simulink model "grabber"  (Simulink 6.4)
settings: Solver=ode45  StartTime=0.0  StopTime=inf  RelTol=1e-3
libraries: vipsnks x1, imaqlib x1
settings Model: LastModifiedBy=usman

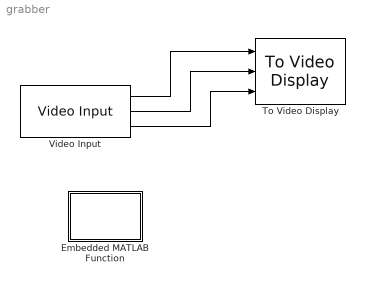
== system grabber ==
  Embedded MATLAB Function : Stateflow chart
  To Video Display : vipsnks/To Video Display  inputType=RGB  OutputDevice=On-screen video monitor  fullScreen=off  videoWindowX=44  videoWindowY=38  saveWindowSize=off  videoWindowWidth=776  videoWindowHeight=606
  Video Input : imaqlib/Video Input  DialogController=imaqcreatedialog  DialogControllerArgs=DataTag0  VideoDeviceMenu=1 (Bt878 TV Card)  VideoDevice=1 (Bt878 TV Card)  VideoStreamFormatMenu=RGB555_768x576  VideoStreamFormat=RGB555_768x576  VideoFrameSize=INPUTSIZE  FrameRate=10 fps  DataType=double
  wires:
  Video Input/1 -> To Video Display/1
  Video Input/2 -> To Video Display/2
  Video Input/3 -> To Video Display/3

== matlab function Embedded MATLAB Function ==
function test
camobject = videoinput ( 'winvideo', 1 )
start ( camobject )
preview ( camobject )
